simulink model "Bank_residuow"  (Simulink 9.1)
settings: Solver=FixedStepAuto  StartTime=0.0  StopTime=1009  FixedStep=0.01  RelTol=1e-8  EnableMultiTasking=on
values from neighbouring files (symbols this model uses):
  G = 4.2    [net_opuznienie_30.mat]    (also in parametrySilnika.m)
  G1 = 4.2    [net_opuznienie_30.mat]    (also in parametrySilnika.m)
  J = 1    [net_opuznienie_30.mat]    (also in parametrySilnika.m)
  J1 = 1.3    [net_opuznienie_30.mat]    (also in parametrySilnika.m = 1)
  Lt = 46    [net_opuznienie_30.mat]    (also in parametrySilnika.m)
  Lt1 = 59.8    [net_opuznienie_30.mat]    (also in parametrySilnika.m = 69)
  Lw = 125    [net_opuznienie_30.mat]    (also in parametrySilnika.m)
  Lw1 = 162.5    [net_opuznienie_30.mat]    (also in parametrySilnika.m = 125)
  Rt = 5    [net_opuznienie_30.mat]    (also in parametrySilnika.m)
  Rt1 = 5    [net_opuznienie_30.mat]    (also in parametrySilnika.m)
undefined symbols (not defined in the file or in its folder): sigbuilder_block
libraries: neural x180, simulink x2
(part 6 of 6)

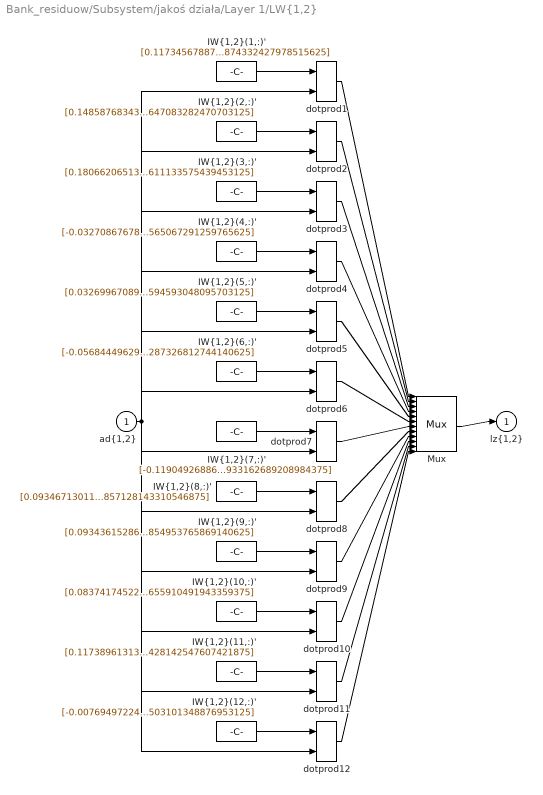
== system Bank_residuow/Subsystem/jakoś działa/Layer 1/LW{1,2} ==
  "ad{1,2}" : Inport  PortDimensions=6  SampleTime=0.1
      mask Display: e = 0.06;c1 = [120 230 180]/255;c2 = ([120 230 180]+0)/(256+128);c3 = ([120 230 180]+128)/(256+128);patch([0 1 1 0],[0 0 1 1],c1);patch([0 1 1 1-e 1-e 0+e],[0 0 1 1-e 0+e 0+e],c2);patch([0 0 1 1-e 0+e 0+e],[0 1 1 1-e 1-e 0+e],c3);plot([0 1 1 0 0],[0 0 1 1 0]);
  "IW{1,2}(1,:)'" : Constant  Value=[0.11734567887645271089258613983474788255989551544189453125;-0.01420744478953828160427974580670706927776336669921875;-0.060957171090602051133355843148819985799491405487060546875;-0.1325684634655676930048429085218231193721294403076171875;-0.0266577004250395932505313112415024079382419586181640625;-0.026971996256349418941145046346719027496874332427978515625]
      mask Display: e = 0.06;c1 = [120 150 230]/255;c2 = ([120 150 230]+0)/383;c3 = ([120 150 230]+128)/383;patch([0 1 1 0],[0 0 1 1],c1);patch([0 1 1 1-e 1-e 0+e],[0 0 1 1-e 0+e 0+e],c2);patch([0 0 1 1-e 0+e 0+e],[0 1 1 1-e 1-e 0+e],c3);plot([0 1 1 0 0],[0 0 1 1 0]);disp('weights');
  "IW{1,2}(10,:)'" : Constant  Value=[0.08374174522886368432494919034070335328578948974609375;0.167657479125779051987166212711599655449390411376953125;-0.2315454931272337424363882973921135999262332916259765625;-0.00635173689870405060176050682230197708122432231903076171875;-0.094810209785529286907745927237556315958499908447265625;0.18106614297742706920502087086788378655910491943359375]
      mask Display: e = 0.06;c1 = [120 150 230]/255;c2 = ([120 150 230]+0)/383;c3 = ([120 150 230]+128)/383;patch([0 1 1 0],[0 0 1 1],c1);patch([0 1 1 1-e 1-e 0+e],[0 0 1 1-e 0+e 0+e],c2);patch([0 0 1 1-e 0+e 0+e],[0 1 1 1-e 1-e 0+e],c3);plot([0 1 1 0 0],[0 0 1 1 0]);disp('weights');
  "IW{1,2}(11,:)'" : Constant  Value=[0.117389613135938153387627380652702413499355316162109375;0.177254423319037790474084204106475226581096649169921875;-0.2502713332598884843349651418975554406642913818359375;0.05814991133562517899857624570358893834054470062255859375;-0.08466366495821732451876329150763922370970249176025390625;0.2112605007851841854016328170473570935428142547607421875]
      mask Display: e = 0.06;c1 = [120 150 230]/255;c2 = ([120 150 230]+0)/383;c3 = ([120 150 230]+128)/383;patch([0 1 1 0],[0 0 1 1],c1);patch([0 1 1 1-e 1-e 0+e],[0 0 1 1-e 0+e 0+e],c2);patch([0 0 1 1-e 0+e 0+e],[0 1 1 1-e 1-e 0+e],c3);plot([0 1 1 0 0],[0 0 1 1 0]);disp('weights');
  "IW{1,2}(12,:)'" : Constant  Value=[-0.007694972249173654375853370623872251599095761775970458984375;-0.10145625910730009244797855672004516236484050750732421875;0.0848581584844336489492633290865342132747173309326171875;0.0819428734153271609574886724658426828682422637939453125;0.17461603454585794548137300807866267859935760498046875;-0.2301237902204789353977076871160534210503101348876953125]
      mask Display: e = 0.06;c1 = [120 150 230]/255;c2 = ([120 150 230]+0)/383;c3 = ([120 150 230]+128)/383;patch([0 1 1 0],[0 0 1 1],c1);patch([0 1 1 1-e 1-e 0+e],[0 0 1 1-e 0+e 0+e],c2);patch([0 0 1 1-e 0+e 0+e],[0 1 1 1-e 1-e 0+e],c3);plot([0 1 1 0 0],[0 0 1 1 0]);disp('weights');
  "IW{1,2}(2,:)'" : Constant  Value=[0.148587683437623130355831335691618733108043670654296875;0.1916398661836554440096591633846401236951351165771484375;0.122732055190232447472453713999129831790924072265625;0.011052955351952505058665821024987963028252124786376953125;-0.066255804787684835499561586402705870568752288818359375;-0.2070439943851332398327969031015527434647083282470703125]
      mask Display: e = 0.06;c1 = [120 150 230]/255;c2 = ([120 150 230]+0)/383;c3 = ([120 150 230]+128)/383;patch([0 1 1 0],[0 0 1 1],c1);patch([0 1 1 1-e 1-e 0+e],[0 0 1 1-e 0+e 0+e],c2);patch([0 0 1 1-e 0+e 0+e],[0 1 1 1-e 1-e 0+e],c3);plot([0 1 1 0 0],[0 0 1 1 0]);disp('weights');
  "IW{1,2}(3,:)'" : Constant  Value=[0.1806620651333467886257011514317127875983715057373046875;-0.303091921515867446235148463529185391962528228759765625;0.08836793314782644126470501078074448741972446441650390625;0.09703643628597248549372267234502942301332950592041015625;0.25615297465495923123768307050340808928012847900390625;-0.1318657253614128610497147064961609430611133575439453125]
      mask Display: e = 0.06;c1 = [120 150 230]/255;c2 = ([120 150 230]+0)/383;c3 = ([120 150 230]+128)/383;patch([0 1 1 0],[0 0 1 1],c1);patch([0 1 1 1-e 1-e 0+e],[0 0 1 1-e 0+e 0+e],c2);patch([0 0 1 1-e 0+e 0+e],[0 1 1 1-e 1-e 0+e],c3);plot([0 1 1 0 0],[0 0 1 1 0]);disp('weights');
  "IW{1,2}(4,:)'" : Constant  Value=[-0.032708676786471831132718790513536077924072742462158203125;-0.07982082665610830407576514744505402632057666778564453125;-0.27182850427708127316606123713427223265171051025390625;0.033260320942053216153322381387624773196876049041748046875;0.1479647247389947739559801220821100287139415740966796875;0.162567678452940234112844564151600934565067291259765625]
      mask Display: e = 0.06;c1 = [120 150 230]/255;c2 = ([120 150 230]+0)/383;c3 = ([120 150 230]+128)/383;patch([0 1 1 0],[0 0 1 1],c1);patch([0 1 1 1-e 1-e 0+e],[0 0 1 1-e 0+e 0+e],c2);patch([0 0 1 1-e 0+e 0+e],[0 1 1 1-e 1-e 0+e],c3);plot([0 1 1 0 0],[0 0 1 1 0]);disp('weights');
  "IW{1,2}(5,:)'" : Constant  Value=[0.032699670897456865892305444276644266210496425628662109375;0.0982811224744134237507608986561535857617855072021484375;0.494758994647634009478309735641232691705226898193359375;-0.016970031549458593211898715935603831894695758819580078125;-0.07631170065071816999147102933420683257281780242919921875;-0.06725314868118570377220066802692599594593048095703125]
      mask Display: e = 0.06;c1 = [120 150 230]/255;c2 = ([120 150 230]+0)/383;c3 = ([120 150 230]+128)/383;patch([0 1 1 0],[0 0 1 1],c1);patch([0 1 1 1-e 1-e 0+e],[0 0 1 1-e 0+e 0+e],c2);patch([0 0 1 1-e 0+e 0+e],[0 1 1 1-e 1-e 0+e],c3);plot([0 1 1 0 0],[0 0 1 1 0]);disp('weights');
  "IW{1,2}(6,:)'" : Constant  Value=[-0.0568444962995343361367162060560076497495174407958984375;0.035835829535056810957183159871419775299727916717529296875;0.26339971114917115624365351322921924293041229248046875;0.0352392221951539352797766468938789330422878265380859375;-0.004276027794509153732993578245213939226232469081878662109375;-0.0757025594573195181880009840824641287326812744140625]
      mask Display: e = 0.06;c1 = [120 150 230]/255;c2 = ([120 150 230]+0)/383;c3 = ([120 150 230]+128)/383;patch([0 1 1 0],[0 0 1 1],c1);patch([0 1 1 1-e 1-e 0+e],[0 0 1 1-e 0+e 0+e],c2);patch([0 0 1 1-e 0+e 0+e],[0 1 1 1-e 1-e 0+e],c3);plot([0 1 1 0 0],[0 0 1 1 0]);disp('weights');
  "IW{1,2}(7,:)'" : Constant  Value=[-0.1190492688632540374538137939453008584678173065185546875;-0.08258118140757599034973424068084568716585636138916015625;-0.36133065563574684464498432134860195219516754150390625;0.087632299447009287529652965531568042933940887451171875;0.062339973433587055062776727254458819516003131866455078125;-0.154340219444939863446819572345702908933162689208984375]
      mask Display: e = 0.06;c1 = [120 150 230]/255;c2 = ([120 150 230]+0)/383;c3 = ([120 150 230]+128)/383;patch([0 1 1 0],[0 0 1 1],c1);patch([0 1 1 1-e 1-e 0+e],[0 0 1 1-e 0+e 0+e],c2);patch([0 0 1 1-e 0+e 0+e],[0 1 1 1-e 1-e 0+e],c3);plot([0 1 1 0 0],[0 0 1 1 0]);disp('weights');
  "IW{1,2}(8,:)'" : Constant  Value=[0.09346713011780861946053988731364370323717594146728515625;0.275115949948501803401512688651564531028270721435546875;0.19430470013122957961826386963366530835628509521484375;-0.04102979127358634403588411032615113072097301483154296875;-0.150601624877191919704699785143020562827587127685546875;-0.2069168630370283590291791142590227536857128143310546875]
      mask Display: e = 0.06;c1 = [120 150 230]/255;c2 = ([120 150 230]+0)/383;c3 = ([120 150 230]+128)/383;patch([0 1 1 0],[0 0 1 1],c1);patch([0 1 1 1-e 1-e 0+e],[0 0 1 1-e 0+e 0+e],c2);patch([0 0 1 1-e 0+e 0+e],[0 1 1 1-e 1-e 0+e],c3);plot([0 1 1 0 0],[0 0 1 1 0]);disp('weights');
  "IW{1,2}(9,:)'" : Constant  Value=[0.09343615286148831966528405246208421885967254638671875;0.10960943996895877727837387283216230571269989013671875;0.450566019832451092330671826857724227011203765869140625;-0.07134394635021452935053076771509950049221515655517578125;-0.07785129982189296915517928709959960542619228363037109375;-0.0046794816202196699850279770771521725691854953765869140625]
      mask Display: e = 0.06;c1 = [120 150 230]/255;c2 = ([120 150 230]+0)/383;c3 = ([120 150 230]+128)/383;patch([0 1 1 0],[0 0 1 1],c1);patch([0 1 1 1-e 1-e 0+e],[0 0 1 1-e 0+e 0+e],c2);patch([0 0 1 1-e 0+e 0+e],[0 1 1 1-e 1-e 0+e],c3);plot([0 1 1 0 0],[0 0 1 1 0]);disp('weights');
  Mux : Mux  Inputs=12
      mask Display: e = 0.06;c1 = [120 150 230]/255;c2 = ([120 150 230]+0)/383;c3 = ([120 150 230]+128)/383;patch([0 1 1 0],[0 0 1 1],c1);patch([0 1 1 1-e 1-e 0+e],[0 0 1 1-e 0+e 0+e],c2);patch([0 0 1 1-e 0+e 0+e],[0 1 1 1-e 1-e 0+e],c3);plot([0 1 1 0 0],[0 0 1 1 0]);disp('Mux');
  dotprod{1..12} (12 alike) : neural/Weight Functions/dotprod
  "lz{1,2}" : Outport
      mask Display: e = 0.06;c1 = [120 230 180]/255;c2 = ([120 230 180]+0)/(256+128);c3 = ([120 230 180]+128)/(256+128);patch([0 1 1 0],[0 0 1 1],c1);patch([0 1 1 1-e 1-e 0+e],[0 0 1 1-e 0+e 0+e],c2);patch([0 0 1 1-e 0+e 0+e],[0 1 1 1-e 1-e 0+e],c3);plot([0 1 1 0 0],[0 0 1 1 0]);
  wires:
  "IW{1,2}(1,:)'"/1 -> dotprod1/1
  "ad{1,2}"/1 -> dotprod1/2, dotprod2/2, dotprod3/2, dotprod4/2, dotprod5/2, dotprod6/2, dotprod7/2, dotprod8/2, dotprod9/2, dotprod10/2, dotprod11/2, dotprod12/2
  dotprod1/1 -> Mux/1
  "IW{1,2}(2,:)'"/1 -> dotprod2/1
  dotprod2/1 -> Mux/2
  "IW{1,2}(3,:)'"/1 -> dotprod3/1
  dotprod3/1 -> Mux/3
  "IW{1,2}(4,:)'"/1 -> dotprod4/1
  dotprod4/1 -> Mux/4
  "IW{1,2}(5,:)'"/1 -> dotprod5/1
  dotprod5/1 -> Mux/5
  "IW{1,2}(6,:)'"/1 -> dotprod6/1
  dotprod6/1 -> Mux/6
  "IW{1,2}(7,:)'"/1 -> dotprod7/1
  dotprod7/1 -> Mux/7
  "IW{1,2}(8,:)'"/1 -> dotprod8/1
  dotprod8/1 -> Mux/8
  "IW{1,2}(9,:)'"/1 -> dotprod9/1
  dotprod9/1 -> Mux/9
  "IW{1,2}(10,:)'"/1 -> dotprod10/1
  dotprod10/1 -> Mux/10
  "IW{1,2}(11,:)'"/1 -> dotprod11/1
  dotprod11/1 -> Mux/11
  "IW{1,2}(12,:)'"/1 -> dotprod12/1
  dotprod12/1 -> Mux/12
  Mux/1 -> "lz{1,2}"/1

== system Bank_residuow/Subsystem/jakoś działa/Layer 2/Delays 1 ==
  "p{2}" : Inport  PortDimensions=12  SampleTime=0.1
      mask Display: e = 0.06;c1 = [120 230 180]/255;c2 = ([120 230 180]+0)/(256+128);c3 = ([120 230 180]+128)/(256+128);patch([0 1 1 0],[0 0 1 1],c1);patch([0 1 1 1-e 1-e 0+e],[0 0 1 1-e 0+e 0+e],c2);patch([0 0 1 1-e 0+e 0+e],[0 1 1 1-e 1-e 0+e],c3);plot([0 1 1 0 0],[0 0 1 1 0]);
  mux : Mux  Inputs=1
      mask Display: e = 0.06;c1 = [120 150 230]/255;c2 = ([120 150 230]+0)/383;c3 = ([120 150 230]+128)/383;patch([0 1 1 0],[0 0 1 1],c1);patch([0 1 1 1-e 1-e 0+e],[0 0 1 1-e 0+e 0+e],c2);patch([0 0 1 1-e 0+e 0+e],[0 1 1 1-e 1-e 0+e],c3);plot([0 1 1 0 0],[0 0 1 1 0]);disp('Mux')
  "pd{2,1}" : Outport
      mask Display: e = 0.06;c1 = [120 230 180]/255;c2 = ([120 230 180]+0)/(256+128);c3 = ([120 230 180]+128)/(256+128);patch([0 1 1 0],[0 0 1 1],c1);patch([0 1 1 1-e 1-e 0+e],[0 0 1 1-e 0+e 0+e],c2);patch([0 0 1 1-e 0+e 0+e],[0 1 1 1-e 1-e 0+e],c3);plot([0 1 1 0 0],[0 0 1 1 0]);
  wires:
  "p{2}"/1 -> mux/1
  mux/1 -> "pd{2,1}"/1

== system Bank_residuow/Subsystem/jakoś działa/Layer 2/LW{2,1} ==
  "ad{2,1}" : Inport  PortDimensions=12  SampleTime=0.1
      mask Display: e = 0.06;c1 = [120 230 180]/255;c2 = ([120 230 180]+0)/(256+128);c3 = ([120 230 180]+128)/(256+128);patch([0 1 1 0],[0 0 1 1],c1);patch([0 1 1 1-e 1-e 0+e],[0 0 1 1-e 0+e 0+e],c2);patch([0 0 1 1-e 0+e 0+e],[0 1 1 1-e 1-e 0+e],c3);plot([0 1 1 0 0],[0 0 1 1 0]);
  "IW{2,1}(1,:)'" : Constant  Value=[1.6306649033456384056961496753501705825328826904296875;0.470468952023564479514305958218756131827831268310546875;2.048311738868989539952281120349653065204620361328125;-0.1661169009458415557478616619846434332430362701416015625;0.459119520954480442309630916497553698718547821044921875;-1.4139618859993756672110976069234311580657958984375;-0.475071720038856504242374967361683957278728485107421875;0.6942384478858112384358491908642463386058807373046875;0.351211322424243466144844205700792372226715087890625;0.69738815967599909750873621305800043046474456787109375;0.92775836594828275938340311768115498125553131103515625;-0.7762362751947147199160781383397988975048065185546875]
      mask Display: e = 0.06;c1 = [120 150 230]/255;c2 = ([120 150 230]+0)/383;c3 = ([120 150 230]+128)/383;patch([0 1 1 0],[0 0 1 1],c1);patch([0 1 1 1-e 1-e 0+e],[0 0 1 1-e 0+e 0+e],c2);patch([0 0 1 1-e 0+e 0+e],[0 1 1 1-e 1-e 0+e],c3);plot([0 1 1 0 0],[0 0 1 1 0]);disp('weights');
  "IW{2,1}(2,:)'" : Constant  Value=[-1.0123076802227906068054608113016001880168914794921875;1.6969419033512114225459299632348120212554931640625;-2.967444134069946670706485747359693050384521484375;1.660862710424467092451550342957489192485809326171875;0.5284640615822338016727144349715672433376312255859375;-0.12197407251094850855199780426119104959070682525634765625;-0.4987961455518894471339308438473381102085113525390625;2.261524331647625896124509381479583680629730224609375;0.53041323736948731148999058859772048890590667724609375;0.925055586862043810469913296401500701904296875;2.085509466259618083228133400552906095981597900390625;1.3472151490065618073543873833841644227504730224609375]
      mask Display: e = 0.06;c1 = [120 150 230]/255;c2 = ([120 150 230]+0)/383;c3 = ([120 150 230]+128)/383;patch([0 1 1 0],[0 0 1 1],c1);patch([0 1 1 1-e 1-e 0+e],[0 0 1 1-e 0+e 0+e],c2);patch([0 0 1 1-e 0+e 0+e],[0 1 1 1-e 1-e 0+e],c3);plot([0 1 1 0 0],[0 0 1 1 0]);disp('weights');
  "IW{2,1}(3,:)'" : Constant  Value=[-0.66130350217804634294083143686293624341487884521484375;0.61516951784502171829416283799218945205211639404296875;0.1944603152843837057250908628702745772898197174072265625;-1.0284740964027465626173807322629727423191070556640625;1.0453858617950906317872750150854699313640594482421875;0.84162373244485932932690275265485979616641998291015625;-0.88862934256105063912656305546988733112812042236328125;0.45667718658935252395991710727685131132602691650390625;1.3045252657808410479134408888057805597782135009765625;-1.403134777643110897571432360564358532428741455078125;-1.0109671795033354779747014617896638810634613037109375;0.73341412022080121335676494709332473576068878173828125]
      mask Display: e = 0.06;c1 = [120 150 230]/255;c2 = ([120 150 230]+0)/383;c3 = ([120 150 230]+128)/383;patch([0 1 1 0],[0 0 1 1],c1);patch([0 1 1 1-e 1-e 0+e],[0 0 1 1-e 0+e 0+e],c2);patch([0 0 1 1-e 0+e 0+e],[0 1 1 1-e 1-e 0+e],c3);plot([0 1 1 0 0],[0 0 1 1 0]);disp('weights');
  Mux : Mux  Inputs=3
      mask Display: e = 0.06;c1 = [120 150 230]/255;c2 = ([120 150 230]+0)/383;c3 = ([120 150 230]+128)/383;patch([0 1 1 0],[0 0 1 1],c1);patch([0 1 1 1-e 1-e 0+e],[0 0 1 1-e 0+e 0+e],c2);patch([0 0 1 1-e 0+e 0+e],[0 1 1 1-e 1-e 0+e],c3);plot([0 1 1 0 0],[0 0 1 1 0]);disp('Mux');
  dotprod1 : neural/Weight Functions/dotprod
  dotprod2 : neural/Weight Functions/dotprod
  dotprod3 : neural/Weight Functions/dotprod
  "lz{2,1}" : Outport
      mask Display: e = 0.06;c1 = [120 230 180]/255;c2 = ([120 230 180]+0)/(256+128);c3 = ([120 230 180]+128)/(256+128);patch([0 1 1 0],[0 0 1 1],c1);patch([0 1 1 1-e 1-e 0+e],[0 0 1 1-e 0+e 0+e],c2);patch([0 0 1 1-e 0+e 0+e],[0 1 1 1-e 1-e 0+e],c3);plot([0 1 1 0 0],[0 0 1 1 0]);
  wires:
  "IW{2,1}(1,:)'"/1 -> dotprod1/1
  "ad{2,1}"/1 -> dotprod1/2, dotprod2/2, dotprod3/2
  dotprod1/1 -> Mux/1
  "IW{2,1}(2,:)'"/1 -> dotprod2/1
  dotprod2/1 -> Mux/2
  "IW{2,1}(3,:)'"/1 -> dotprod3/1
  dotprod3/1 -> Mux/3
  Mux/1 -> "lz{2,1}"/1
